simulink model "minseg_M2V3_2017a"  (R2017a)
settings: Solver=FixedStepDiscrete  StartTime=0.0  StopTime=inf  FixedStep=mdl_T_sample  RelTol=1e-3
undefined symbols (not defined in the file or in its folder): ctrl_lqr_K2, ctrl_motorDriver_v_ff_cmd_v_val, ctrl_motorDriver_v_ff_cmd_v_val_norm_dx_max, ctrl_motorDriver_v_ff_cmd_v_val_norm_dx_min, ctrl_motorDriver_v_output_max, ctrl_motorDriver_v_output_min, ctrl_motorDriver_v_pid_cmd_thetaDot_val, ctrl_motorDriver_v_pid_cmd_thetaDot_val_norm_dx_max, ctrl_motorDriver_v_pid_cmd_thetaDot_val_norm_dx_min, ctrl_motorDriver_v_pid_int_maxVal, ctrl_motorDriver_v_pid_int_minVal, ctrl_motorDriver_v_pid_k_d, ctrl_motorDriver_v_pid_k_i, ctrl_motorDriver_v_pid_k_p, ctrl_motorDriver_v_rts_ss_k_A, ctrl_motorDriver_v_rts_ss_k_B, ctrl_motorDriver_v_rts_ss_k_C, ctrl_motorDriver_v_rts_ss_k_D, ctrl_motorDriver_v_rts_ss_stateIC, ctrl_motorDriver_v_sfr_cmd_p_x_f, ctrl_motorDriver_v_sfr_cmd_p_x_mag, ctrl_motorDriver_v_sfr_cmd_p_y_f, ctrl_motorDriver_v_sfr_cmd_p_y_mag, ctrl_motorDriver_v_sfr_K, ctrl_motorDriver_v_sfr_K_plant, ctrl_motorDriver_v_sfr_K_rts, ctrl_motorDriver_v_T_cmd, ctrl_motorDriver_v_T_init, DiscIntNeverNeededParam, gyro_bias, io_srl_read_rateTransition_initialCondition, k_intmax_uint8, mdl_T_sample, mtr_encoder_filter_z_ss_A, mtr_encoder_filter_z_ss_B, mtr_encoder_filter_z_ss_C, mtr_encoder_filter_z_ss_D, plant, plant_accel_k_digital2analog, plant_body_l_c, plant_body_l_w, plant_gyro_encoder_filter_z_den, plant_gyro_encoder_filter_z_num, plant_gyro_filter_z_den, plant_gyro_filter_z_num, plant_gyro_k_digital2analog, plant_linear_ss_stateIC, plant_linear_ss_t_A, plant_linear_ss_t_B, plant_linear_ss_t_C, plant_linear_ss_t_D, plant_mtr_encoder_count2wheelRad, plant_mtr_encoder_filter_z_den, plant_mtr_encoder_filter_z_num, plant_pSupply_v, plant_supply_v, plant_T_init, plant_wheel_r
undefined symbols (not defined in the file): ctrl_lqr_addlDyn_A_discrete, ctrl_lqr_addlDyn_B_discrete, ctrl_lqr_addlDyn_C_discrete, ctrl_lqr_addlDyn_D_discrete, ctrl_lqr_addlDyn_k_antiWindup, ctrl_lqr_addlDyn_stateIC, plant_gyro_bias_movingAverage_n_pts, plant_linear_A_continuous, plant_linear_B_continuous, plant_linear_C_continuous, plant_linear_D_continuous, plant_linear_stateIC
libraries: svdutilitieslib x135, simulink x57, arduinolib x15, MinSegLibrary_M2V3 x3, dspindex x3, RASPlib x2
(part 4 of 6)

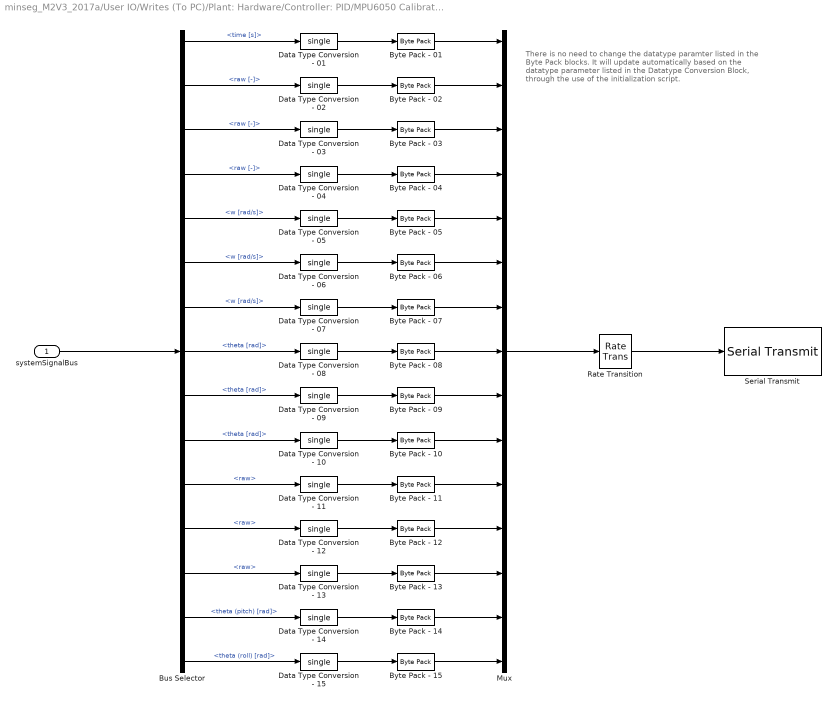
== system minseg_M2V3_2017a/User IO/Writes (To PC)/Plant: Hardware/Controller: PID/MPU6050 Calibration ==
  note: There is no need to change the datatype paramter
      | listed in the Byte Pack blocks.
      |
      | It will update automatically based on the datatype parameter
      | listed in the Datatype Conversion Block,
      | through the use of the initialization script.
  systemSignalBus : Inport
  Bus Selector : BusSelector  OutputSignals=plant.clock.time [s],plant.gyroscope.x.raw [-],plant.gyroscope.y.raw [-],plant.gyroscope.z.raw [-],plant.gyroscope.x.w [rad/s],plant.gyroscope.y.w [rad/s],plant.gyroscope.z.w [rad/s],plant.gyroscope.x.theta [rad],plant.gyroscope.y.theta [rad],plant.gyroscope.z.theta [rad],plant.accelerometer.x.raw,plant.accelerometer.y.raw,plant.accelerometer.z.raw,plant.accelerometer.x.theta (pitch) [rad],plant.accelerometer.z.theta (roll) [rad]
  Byte Pack - 01 : svdutilitieslib/Byte Pack  datatypes={'single'}  byteAlign=1  blockPlatform=arduinoert
      settings: AttributesFormatString=%<datatypes>  SourceProductName=Simulink Support Package for Arduino Hardware
  Byte Pack - 02 : svdutilitieslib/Byte Pack  datatypes={'single'}  byteAlign=1  blockPlatform=arduinoert
      settings: AttributesFormatString=%<datatypes>  SourceProductName=Simulink Support Package for Arduino Hardware
  Byte Pack - 03 : svdutilitieslib/Byte Pack  datatypes={'single'}  byteAlign=1  blockPlatform=arduinoert
      settings: AttributesFormatString=%<datatypes>  SourceProductName=Simulink Support Package for Arduino Hardware
  Byte Pack - 04 : svdutilitieslib/Byte Pack  datatypes={'single'}  byteAlign=1  blockPlatform=arduinoert
      settings: AttributesFormatString=%<datatypes>  SourceProductName=Simulink Support Package for Arduino Hardware
  Byte Pack - 05 : svdutilitieslib/Byte Pack  datatypes={'single'}  byteAlign=1  blockPlatform=arduinoert
      settings: AttributesFormatString=%<datatypes>  SourceProductName=Simulink Support Package for Arduino Hardware
  Byte Pack - 06 : svdutilitieslib/Byte Pack  datatypes={'single'}  byteAlign=1  blockPlatform=arduinoert
      settings: AttributesFormatString=%<datatypes>  SourceProductName=Simulink Support Package for Arduino Hardware
  Byte Pack - 07 : svdutilitieslib/Byte Pack  datatypes={'single'}  byteAlign=1  blockPlatform=arduinoert
      settings: AttributesFormatString=%<datatypes>  SourceProductName=Simulink Support Package for Arduino Hardware
  Byte Pack - 08 : svdutilitieslib/Byte Pack  datatypes={'single'}  byteAlign=1  blockPlatform=arduinoert
      settings: AttributesFormatString=%<datatypes>  SourceProductName=Simulink Support Package for Arduino Hardware
  Byte Pack - 09 : svdutilitieslib/Byte Pack  datatypes={'single'}  byteAlign=1  blockPlatform=arduinoert
      settings: AttributesFormatString=%<datatypes>  SourceProductName=Simulink Support Package for Arduino Hardware
  Byte Pack - {10..15} (6 alike) : svdutilitieslib/Byte Pack  datatypes={'single'}  byteAlign=1  blockPlatform=arduinoert
      settings: AttributesFormatString=%<datatypes>  SourceProductName=Simulink Support Package for Arduino Hardware
  Data Type Conversion - 01 : DataTypeConversion  OutDataTypeStr=single
  Data Type Conversion - 02 : DataTypeConversion  OutDataTypeStr=single
  Data Type Conversion - 03 : DataTypeConversion  OutDataTypeStr=single
  Data Type Conversion - 04 : DataTypeConversion  OutDataTypeStr=single
  Data Type Conversion - 05 : DataTypeConversion  OutDataTypeStr=single
  Data Type Conversion - 06 : DataTypeConversion  OutDataTypeStr=single
  Data Type Conversion - 07 : DataTypeConversion  OutDataTypeStr=single
  Data Type Conversion - 08 : DataTypeConversion  OutDataTypeStr=single
  Data Type Conversion - 09 : DataTypeConversion  OutDataTypeStr=single
  Data Type Conversion - {10..15} (6 alike) : DataTypeConversion  OutDataTypeStr=single
  Mux : Mux  Inputs=15
  Rate Transition : RateTransition  X0=io_srl_read_rateTransition_initialCondition  OutPortSampleTimeMultiple=io_read_rateTransition_decimation  OutPortSampleTime=io_srl_read_rateTransition_T_sample
      settings: AttributesFormatString=|
      | Output sample time: %<OutPortSampleTime>
      | Initial condition: %<X0>
  Serial Transmit : arduinolib/Serial Transmit  portNumber=0  sendmode=write  sendformat=Decimal  floatprecision=2  blockPlatform=arduino
      settings: SourceProductName=Simulink Support Package for Arduino Hardware
  wires:
  Byte Pack - 04/1 -> Mux/4
  Byte Pack - 03/1 -> Mux/3
  Byte Pack - 07/1 -> Mux/7
  Mux/1 -> Rate Transition/1
  Byte Pack - 01/1 -> Mux/1
  Byte Pack - 06/1 -> Mux/6
  Byte Pack - 05/1 -> Mux/5
  Byte Pack - 08/1 -> Mux/8
  Byte Pack - 02/1 -> Mux/2
  systemSignalBus/1 -> Bus Selector/1
  Byte Pack - 09/1 -> Mux/9
  Byte Pack - 10/1 -> Mux/10
  Data Type Conversion - 01/1 -> Byte Pack - 01/1
  Data Type Conversion - 02/1 -> Byte Pack - 02/1
  Data Type Conversion - 03/1 -> Byte Pack - 03/1
  Data Type Conversion - 04/1 -> Byte Pack - 04/1
  Data Type Conversion - 05/1 -> Byte Pack - 05/1
  Data Type Conversion - 06/1 -> Byte Pack - 06/1
  Data Type Conversion - 07/1 -> Byte Pack - 07/1
  Data Type Conversion - 08/1 -> Byte Pack - 08/1
  Data Type Conversion - 09/1 -> Byte Pack - 09/1
  Data Type Conversion - 10/1 -> Byte Pack - 10/1
  Rate Transition/1 -> Serial Transmit/1
  Bus Selector/1 -> Data Type Conversion - 01/1  "<time [s]>"
  Data Type Conversion - 11/1 -> Byte Pack - 11/1
  Data Type Conversion - 12/1 -> Byte Pack - 12/1
  Data Type Conversion - 13/1 -> Byte Pack - 13/1
  Data Type Conversion - 14/1 -> Byte Pack - 14/1
  Data Type Conversion - 15/1 -> Byte Pack - 15/1
  Byte Pack - 11/1 -> Mux/11
  Byte Pack - 12/1 -> Mux/12
  Byte Pack - 13/1 -> Mux/13
  Byte Pack - 14/1 -> Mux/14
  Byte Pack - 15/1 -> Mux/15
  Bus Selector/2 -> Data Type Conversion - 02/1  "<raw [-]>"
  Bus Selector/3 -> Data Type Conversion - 03/1  "<raw [-]>"
  Bus Selector/4 -> Data Type Conversion - 04/1  "<raw [-]>"
  Bus Selector/5 -> Data Type Conversion - 05/1  "<w [rad/s]>"
  Bus Selector/6 -> Data Type Conversion - 06/1  "<w [rad/s]>"
  Bus Selector/7 -> Data Type Conversion - 07/1  "<w [rad/s]>"
  Bus Selector/8 -> Data Type Conversion - 08/1  "<theta [rad]>"
  Bus Selector/11 -> Data Type Conversion - 11/1  "<raw>"
  Bus Selector/12 -> Data Type Conversion - 12/1  "<raw>"
  Bus Selector/9 -> Data Type Conversion - 09/1  "<theta [rad]>"
  Bus Selector/10 -> Data Type Conversion - 10/1  "<theta [rad]>"
  Bus Selector/13 -> Data Type Conversion - 13/1  "<raw>"
  Bus Selector/14 -> Data Type Conversion - 14/1  "<theta (pitch) [rad]>"
  Bus Selector/15 -> Data Type Conversion - 15/1  "<theta (roll) [rad]>"

== system minseg_M2V3_2017a/User IO/Writes (To PC)/Plant: Hardware/Controller: PID/Standard ==
  note: There is no need to change the datatype parameter
      | listed in the Byte Pack blocks.
      |
      | It will update automatically based on the datatype parameter
      | listed in the Datatype Conversion Block,
      | through the use of the initialization script.
  systemSignalBus : Inport
  Bus Selector : BusSelector  OutputSignals=clock.time [s],userIO.read.controller.command.left.theta_global_average_dot [rad/s],controller.v_motorDriver.output.left.command [V].saturated,controller.v_motorDriver.output.middle.command [V].saturated,plant.state.wheel_angularPosition_theta_global_average [rad],plant.state.body_angularPosition_phi_x [rad],plant.state.wheel_angularVelocity_thetaDot_global_average [rad/s],plant.state.body_angularVelocity_phiDot_x [rad/s],plant.state.body_angularPosition_phi_y [rad],plant.state.body_angularVelocity_phiDot_y [rad/s]
  Byte Pack - 01 : svdutilitieslib/Byte Pack  datatypes={'single'}  byteAlign=1  blockPlatform=arduinoert
      settings: AttributesFormatString=%<datatypes>  SourceProductName=Simulink Support Package for Arduino Hardware
  Byte Pack - 02 : svdutilitieslib/Byte Pack  datatypes={'single'}  byteAlign=1  blockPlatform=arduinoert
      settings: AttributesFormatString=%<datatypes>  SourceProductName=Simulink Support Package for Arduino Hardware
  Byte Pack - 03 : svdutilitieslib/Byte Pack  datatypes={'single'}  byteAlign=1  blockPlatform=arduinoert
      settings: AttributesFormatString=%<datatypes>  SourceProductName=Simulink Support Package for Arduino Hardware
  Byte Pack - 04 : svdutilitieslib/Byte Pack  datatypes={'single'}  byteAlign=1  blockPlatform=arduinoert
      settings: AttributesFormatString=%<datatypes>  SourceProductName=Simulink Support Package for Arduino Hardware
  Byte Pack - 05 : svdutilitieslib/Byte Pack  datatypes={'single'}  byteAlign=1  blockPlatform=arduinoert
      settings: AttributesFormatString=%<datatypes>  SourceProductName=Simulink Support Package for Arduino Hardware
  Byte Pack - 06 : svdutilitieslib/Byte Pack  datatypes={'single'}  byteAlign=1  blockPlatform=arduinoert
      settings: AttributesFormatString=%<datatypes>  SourceProductName=Simulink Support Package for Arduino Hardware
  Byte Pack - 07 : svdutilitieslib/Byte Pack  datatypes={'single'}  byteAlign=1  blockPlatform=arduinoert
      settings: AttributesFormatString=%<datatypes>  SourceProductName=Simulink Support Package for Arduino Hardware
  Byte Pack - 08 : svdutilitieslib/Byte Pack  datatypes={'single'}  byteAlign=1  blockPlatform=arduinoert
      settings: AttributesFormatString=%<datatypes>  SourceProductName=Simulink Support Package for Arduino Hardware
  Byte Pack - 09 : svdutilitieslib/Byte Pack  datatypes={'single'}  byteAlign=1  blockPlatform=arduinoert
      settings: AttributesFormatString=%<datatypes>  SourceProductName=Simulink Support Package for Arduino Hardware
  Byte Pack - 10 : svdutilitieslib/Byte Pack  datatypes={'single'}  byteAlign=1  blockPlatform=arduinoert
      settings: AttributesFormatString=%<datatypes>  SourceProductName=Simulink Support Package for Arduino Hardware
  Data Type Conversion - 01 : DataTypeConversion  OutDataTypeStr=single
  Data Type Conversion - 02 : DataTypeConversion  OutDataTypeStr=single
  Data Type Conversion - 03 : DataTypeConversion  OutDataTypeStr=single
  Data Type Conversion - 04 : DataTypeConversion  OutDataTypeStr=single
  Data Type Conversion - 05 : DataTypeConversion  OutDataTypeStr=single
  Data Type Conversion - 06 : DataTypeConversion  OutDataTypeStr=single
  Data Type Conversion - 07 : DataTypeConversion  OutDataTypeStr=single
  Data Type Conversion - 08 : DataTypeConversion  OutDataTypeStr=single
  Data Type Conversion - 09 : DataTypeConversion  OutDataTypeStr=single
  Data Type Conversion - 10 : DataTypeConversion  OutDataTypeStr=single
  Mux : Mux  Inputs=10
  Rate Transition : RateTransition  X0=0 %io_srl_read_rateTransition_initialCondition  OutPortSampleTimeMultiple=io_read_rateTransition_decimation  OutPortSampleTime=io_srl_read_rateTransition_T_sample
      settings: AttributesFormatString=|
      | Output sample time: %<OutPortSampleTime>
      | Initial condition: %<X0>
  Serial Transmit : arduinolib/Serial Transmit  portNumber=srl_port  sendmode=write  sendformat=Decimal  floatprecision=2  blockPlatform=arduino
      settings: SourceProductName=Simulink Support Package for Arduino Hardware
  wires:
  Mux/1 -> Serial Transmit/1
  Data Type Conversion - 10/1 -> Byte Pack - 10/1
  Data Type Conversion - 09/1 -> Byte Pack - 09/1
  Data Type Conversion - 08/1 -> Byte Pack - 08/1
  Data Type Conversion - 07/1 -> Byte Pack - 07/1
  Data Type Conversion - 06/1 -> Byte Pack - 06/1
  Data Type Conversion - 05/1 -> Byte Pack - 05/1
  Data Type Conversion - 04/1 -> Byte Pack - 04/1
  Data Type Conversion - 03/1 -> Byte Pack - 03/1
  Data Type Conversion - 02/1 -> Byte Pack - 02/1
  Data Type Conversion - 01/1 -> Byte Pack - 01/1
  Byte Pack - 10/1 -> Mux/10
  Byte Pack - 09/1 -> Mux/9
  systemSignalBus/1 -> Rate Transition/1
  Byte Pack - 02/1 -> Mux/2
  Byte Pack - 08/1 -> Mux/8
  Byte Pack - 05/1 -> Mux/5
  Byte Pack - 06/1 -> Mux/6
  Byte Pack - 01/1 -> Mux/1
  Byte Pack - 07/1 -> Mux/7
  Byte Pack - 03/1 -> Mux/3
  Byte Pack - 04/1 -> Mux/4
  Bus Selector/1 -> Data Type Conversion - 01/1  "<time [s]>"
  Bus Selector/2 -> Data Type Conversion - 02/1  "<theta_global_average_dot [rad/s]>"
  Bus Selector/3 -> Data Type Conversion - 03/1  "<saturated>"
  Bus Selector/4 -> Data Type Conversion - 04/1  "<saturated>"
  Bus Selector/5 -> Data Type Conversion - 05/1  "<wheel_angularPosition_theta_global_average [rad]>"
  Bus Selector/6 -> Data Type Conversion - 06/1  "<body_angularPosition_phi_x [rad]>"
  Bus Selector/7 -> Data Type Conversion - 07/1  "<wheel_angularVelocity_thetaDot_global_average [rad/s]>"
  Bus Selector/8 -> Data Type Conversion - 08/1  "<body_angularVelocity_phiDot_x [rad/s]>"
  Bus Selector/9 -> Data Type Conversion - 09/1  "<body_angularPosition_phi_y [rad]>"
  Bus Selector/10 -> Data Type Conversion - 10/1  "<body_angularVelocity_phiDot_y [rad/s]>"
  Rate Transition/1 -> Bus Selector/1

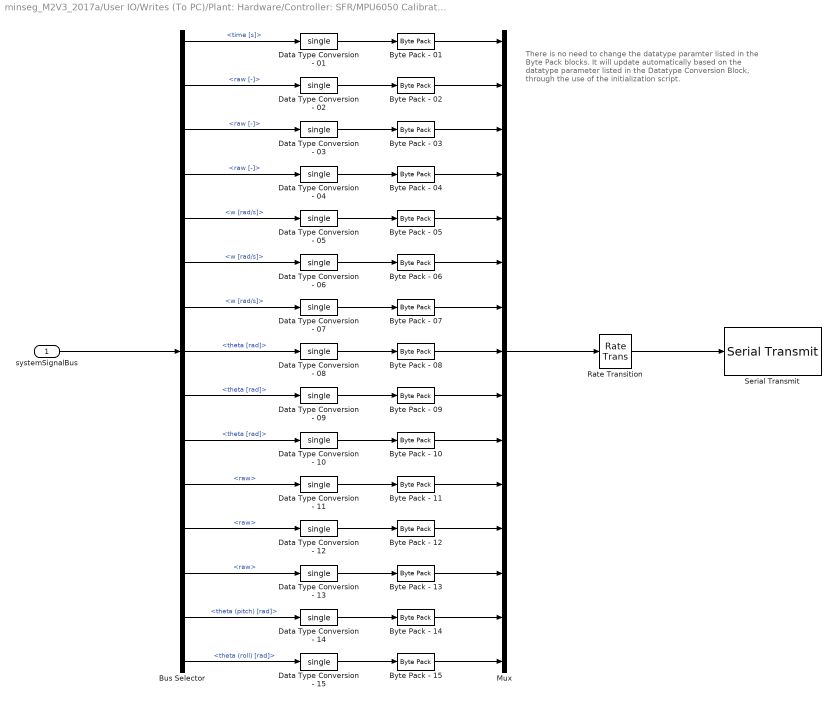
== system minseg_M2V3_2017a/User IO/Writes (To PC)/Plant: Hardware/Controller: SFR/MPU6050 Calibration ==
  note: There is no need to change the datatype paramter
      | listed in the Byte Pack blocks.
      |
      | It will update automatically based on the datatype parameter
      | listed in the Datatype Conversion Block,
      | through the use of the initialization script.
  systemSignalBus : Inport
  Bus Selector : BusSelector  OutputSignals=plant.clock.time [s],plant.gyroscope.x.raw [-],plant.gyroscope.y.raw [-],plant.gyroscope.z.raw [-],plant.gyroscope.x.w [rad/s],plant.gyroscope.y.w [rad/s],plant.gyroscope.z.w [rad/s],plant.gyroscope.x.theta [rad],plant.gyroscope.y.theta [rad],plant.gyroscope.z.theta [rad],plant.accelerometer.x.raw,plant.accelerometer.y.raw,plant.accelerometer.z.raw,plant.accelerometer.x.theta (pitch) [rad],plant.accelerometer.z.theta (roll) [rad]
  Byte Pack - 01 : svdutilitieslib/Byte Pack  datatypes={'single'}  byteAlign=1  blockPlatform=arduinoert
      settings: AttributesFormatString=%<datatypes>  SourceProductName=Simulink Support Package for Arduino Hardware
  Byte Pack - 02 : svdutilitieslib/Byte Pack  datatypes={'single'}  byteAlign=1  blockPlatform=arduinoert
      settings: AttributesFormatString=%<datatypes>  SourceProductName=Simulink Support Package for Arduino Hardware
  Byte Pack - 03 : svdutilitieslib/Byte Pack  datatypes={'single'}  byteAlign=1  blockPlatform=arduinoert
      settings: AttributesFormatString=%<datatypes>  SourceProductName=Simulink Support Package for Arduino Hardware
  Byte Pack - 04 : svdutilitieslib/Byte Pack  datatypes={'single'}  byteAlign=1  blockPlatform=arduinoert
      settings: AttributesFormatString=%<datatypes>  SourceProductName=Simulink Support Package for Arduino Hardware
  Byte Pack - 05 : svdutilitieslib/Byte Pack  datatypes={'single'}  byteAlign=1  blockPlatform=arduinoert
      settings: AttributesFormatString=%<datatypes>  SourceProductName=Simulink Support Package for Arduino Hardware
  Byte Pack - 06 : svdutilitieslib/Byte Pack  datatypes={'single'}  byteAlign=1  blockPlatform=arduinoert
      settings: AttributesFormatString=%<datatypes>  SourceProductName=Simulink Support Package for Arduino Hardware
  Byte Pack - 07 : svdutilitieslib/Byte Pack  datatypes={'single'}  byteAlign=1  blockPlatform=arduinoert
      settings: AttributesFormatString=%<datatypes>  SourceProductName=Simulink Support Package for Arduino Hardware
  Byte Pack - 08 : svdutilitieslib/Byte Pack  datatypes={'single'}  byteAlign=1  blockPlatform=arduinoert
      settings: AttributesFormatString=%<datatypes>  SourceProductName=Simulink Support Package for Arduino Hardware
  Byte Pack - 09 : svdutilitieslib/Byte Pack  datatypes={'single'}  byteAlign=1  blockPlatform=arduinoert
      settings: AttributesFormatString=%<datatypes>  SourceProductName=Simulink Support Package for Arduino Hardware
  Byte Pack - {10..15} (6 alike) : svdutilitieslib/Byte Pack  datatypes={'single'}  byteAlign=1  blockPlatform=arduinoert
      settings: AttributesFormatString=%<datatypes>  SourceProductName=Simulink Support Package for Arduino Hardware
  Data Type Conversion - 01 : DataTypeConversion  OutDataTypeStr=single
  Data Type Conversion - 02 : DataTypeConversion  OutDataTypeStr=single
  Data Type Conversion - 03 : DataTypeConversion  OutDataTypeStr=single
  Data Type Conversion - 04 : DataTypeConversion  OutDataTypeStr=single
  Data Type Conversion - 05 : DataTypeConversion  OutDataTypeStr=single
  Data Type Conversion - 06 : DataTypeConversion  OutDataTypeStr=single
  Data Type Conversion - 07 : DataTypeConversion  OutDataTypeStr=single
  Data Type Conversion - 08 : DataTypeConversion  OutDataTypeStr=single
  Data Type Conversion - 09 : DataTypeConversion  OutDataTypeStr=single
  Data Type Conversion - {10..15} (6 alike) : DataTypeConversion  OutDataTypeStr=single
  Mux : Mux  Inputs=15
  Rate Transition : RateTransition  X0=io_srl_read_rateTransition_initialCondition  OutPortSampleTimeMultiple=io_read_rateTransition_decimation  OutPortSampleTime=io_srl_read_rateTransition_T_sample
      settings: AttributesFormatString=|
      | Output sample time: %<OutPortSampleTime>
      | Initial condition: %<X0>
  Serial Transmit : arduinolib/Serial Transmit  portNumber=0  sendmode=write  sendformat=Decimal  floatprecision=2  blockPlatform=arduino
      settings: SourceProductName=Simulink Support Package for Arduino Hardware
  wires:
  Bus Selector/15 -> Data Type Conversion - 15/1  "<theta (roll) [rad]>"
  Bus Selector/14 -> Data Type Conversion - 14/1  "<theta (pitch) [rad]>"
  Bus Selector/13 -> Data Type Conversion - 13/1  "<raw>"
  Bus Selector/10 -> Data Type Conversion - 10/1  "<theta [rad]>"
  Bus Selector/9 -> Data Type Conversion - 09/1  "<theta [rad]>"
  Bus Selector/12 -> Data Type Conversion - 12/1  "<raw>"
  Bus Selector/11 -> Data Type Conversion - 11/1  "<raw>"
  Bus Selector/8 -> Data Type Conversion - 08/1  "<theta [rad]>"
  Bus Selector/7 -> Data Type Conversion - 07/1  "<w [rad/s]>"
  Bus Selector/6 -> Data Type Conversion - 06/1  "<w [rad/s]>"
  Bus Selector/5 -> Data Type Conversion - 05/1  "<w [rad/s]>"
  Bus Selector/4 -> Data Type Conversion - 04/1  "<raw [-]>"
  Bus Selector/3 -> Data Type Conversion - 03/1  "<raw [-]>"
  Bus Selector/2 -> Data Type Conversion - 02/1  "<raw [-]>"
  Byte Pack - 15/1 -> Mux/15
  Byte Pack - 14/1 -> Mux/14
  Byte Pack - 13/1 -> Mux/13
  Byte Pack - 12/1 -> Mux/12
  Byte Pack - 11/1 -> Mux/11
  Data Type Conversion - 15/1 -> Byte Pack - 15/1
  Data Type Conversion - 14/1 -> Byte Pack - 14/1
  Data Type Conversion - 13/1 -> Byte Pack - 13/1
  Data Type Conversion - 12/1 -> Byte Pack - 12/1
  Data Type Conversion - 11/1 -> Byte Pack - 11/1
  Bus Selector/1 -> Data Type Conversion - 01/1  "<time [s]>"
  Rate Transition/1 -> Serial Transmit/1
  Data Type Conversion - 10/1 -> Byte Pack - 10/1
  Data Type Conversion - 09/1 -> Byte Pack - 09/1
  Data Type Conversion - 08/1 -> Byte Pack - 08/1
  Data Type Conversion - 07/1 -> Byte Pack - 07/1
  Data Type Conversion - 06/1 -> Byte Pack - 06/1
  Data Type Conversion - 05/1 -> Byte Pack - 05/1
  Data Type Conversion - 04/1 -> Byte Pack - 04/1
  Data Type Conversion - 03/1 -> Byte Pack - 03/1
  Data Type Conversion - 02/1 -> Byte Pack - 02/1
  Data Type Conversion - 01/1 -> Byte Pack - 01/1
  Byte Pack - 10/1 -> Mux/10
  Byte Pack - 09/1 -> Mux/9
  systemSignalBus/1 -> Bus Selector/1
  Byte Pack - 02/1 -> Mux/2
  Byte Pack - 08/1 -> Mux/8
  Byte Pack - 05/1 -> Mux/5
  Byte Pack - 06/1 -> Mux/6
  Byte Pack - 01/1 -> Mux/1
  Mux/1 -> Rate Transition/1
  Byte Pack - 07/1 -> Mux/7
  Byte Pack - 03/1 -> Mux/3
  Byte Pack - 04/1 -> Mux/4

== system minseg_M2V3_2017a/User IO/Writes (To PC)/Plant: Hardware/Controller: SFR/Motor Characterization ==
  note: There is no need to change the datatype paramter
      | listed in the Byte Pack blocks.
      |
      | It will update automatically based on the datatype parameter
      | listed in the Datatype Conversion Block,
      | through the use of the initialization script.
  systemSignalBus : Inport
  Bus Selector : BusSelector  OutputSignals="plant.clock.time [s],io.reads.userInput.controller.output_vMotor.command,plant.encoders.left.angularVelocity  [rad/s],plant.encoders.middle.angularVelocity  [rad/s],controller.motorAngularVelocity.left.voltage.command [V],controller.motorAngularVelocity.middle.voltage.command [V],plant.drivers.left.voltage.command.digital.positive [V],plant.drivers.left.voltage.command.digital.negative [V],plant.drivers.middle.voltage.command.digital.positive [V],plant.drivers.middle.voltage.command.digital.negative [V]"
  Byte Pack - 01 : svdutilitieslib/Byte Pack  datatypes={'single'}  byteAlign=1  blockPlatform=arduinoert
      settings: AttributesFormatString=%<datatypes>  SourceProductName=Simulink Support Package for Arduino Hardware
  Byte Pack - 02 : svdutilitieslib/Byte Pack  datatypes={'single'}  byteAlign=1  blockPlatform=arduinoert
      settings: AttributesFormatString=%<datatypes>  SourceProductName=Simulink Support Package for Arduino Hardware
  Byte Pack - 03 : svdutilitieslib/Byte Pack  datatypes={'single'}  byteAlign=1  blockPlatform=arduinoert
      settings: AttributesFormatString=%<datatypes>  SourceProductName=Simulink Support Package for Arduino Hardware
  Byte Pack - 04 : svdutilitieslib/Byte Pack  datatypes={'single'}  byteAlign=1  blockPlatform=arduinoert
      settings: AttributesFormatString=%<datatypes>  SourceProductName=Simulink Support Package for Arduino Hardware
  Byte Pack - 05 : svdutilitieslib/Byte Pack  datatypes={'single'}  byteAlign=1  blockPlatform=arduinoert
      settings: AttributesFormatString=%<datatypes>  SourceProductName=Simulink Support Package for Arduino Hardware
  Byte Pack - 06 : svdutilitieslib/Byte Pack  datatypes={'single'}  byteAlign=1  blockPlatform=arduinoert
      settings: AttributesFormatString=%<datatypes>  SourceProductName=Simulink Support Package for Arduino Hardware
  Byte Pack - 07 : svdutilitieslib/Byte Pack  datatypes={'single'}  byteAlign=1  blockPlatform=arduinoert
      settings: AttributesFormatString=%<datatypes>  SourceProductName=Simulink Support Package for Arduino Hardware
  Byte Pack - 08 : svdutilitieslib/Byte Pack  datatypes={'single'}  byteAlign=1  blockPlatform=arduinoert
      settings: AttributesFormatString=%<datatypes>  SourceProductName=Simulink Support Package for Arduino Hardware
  Byte Pack - 09 : svdutilitieslib/Byte Pack  datatypes={'uint8'}  byteAlign=1  blockPlatform=arduinoert
      settings: AttributesFormatString=%<datatypes>  SourceProductName=Simulink Support Package for Arduino Hardware
  Byte Pack - 10 : svdutilitieslib/Byte Pack  datatypes={'uint8'}  byteAlign=1  blockPlatform=arduinoert
      settings: AttributesFormatString=%<datatypes>  SourceProductName=Simulink Support Package for Arduino Hardware
  Data Type Conversion - 01 : DataTypeConversion  OutDataTypeStr=single
  Data Type Conversion - 02 : DataTypeConversion  OutDataTypeStr=single
  Data Type Conversion - 03 : DataTypeConversion  OutDataTypeStr=single
  Data Type Conversion - 04 : DataTypeConversion  OutDataTypeStr=single
  Data Type Conversion - 05 : DataTypeConversion  OutDataTypeStr=single
  Data Type Conversion - 06 : DataTypeConversion  OutDataTypeStr=single
  Data Type Conversion - 07 : DataTypeConversion  OutDataTypeStr=uint8
  Data Type Conversion - 08 : DataTypeConversion  OutDataTypeStr=uint8
  Data Type Conversion - 09 : DataTypeConversion  OutDataTypeStr=uint8
  Data Type Conversion - 10 : DataTypeConversion  OutDataTypeStr=uint8
  Mux : Mux  Inputs=10
  Rate Transition : RateTransition  X0=io_srl_read_rateTransition_initialCondition  OutPortSampleTimeMultiple=io_read_rateTransition_decimation  OutPortSampleTime=io_srl_read_rateTransition_T_sample
      settings: AttributesFormatString=|
      | Output sample time: %<OutPortSampleTime>
      | Initial condition: %<X0>
  Serial Transmit : arduinolib/Serial Transmit  portNumber=0  sendmode=write  sendformat=Decimal  floatprecision=2  blockPlatform=arduino
      settings: SourceProductName=Simulink Support Package for Arduino Hardware
  wires:
  Bus Selector/10 -> Data Type Conversion - 10/1  "<negative [V]>"
  Bus Selector/9 -> Data Type Conversion - 09/1  "<positive [V]>"
  Bus Selector/8 -> Data Type Conversion - 08/1  "<negative [V]>"
  Bus Selector/7 -> Data Type Conversion - 07/1  "<positive [V]>"
  Bus Selector/6 -> Data Type Conversion - 06/1  "<command [V]>"
  Bus Selector/5 -> Data Type Conversion - 05/1  "<command [V]>"
  Byte Pack - 04/1 -> Mux/4
  Byte Pack - 03/1 -> Mux/3
  Byte Pack - 07/1 -> Mux/7
  Mux/1 -> Rate Transition/1
  Byte Pack - 01/1 -> Mux/1
  Byte Pack - 06/1 -> Mux/6
  Byte Pack - 05/1 -> Mux/5
  Byte Pack - 08/1 -> Mux/8
  Byte Pack - 02/1 -> Mux/2
  systemSignalBus/1 -> Bus Selector/1
  Bus Selector/2 -> Data Type Conversion - 02/1  "<command>"
  Byte Pack - 09/1 -> Mux/9
  Byte Pack - 10/1 -> Mux/10
  Data Type Conversion - 01/1 -> Byte Pack - 01/1
  Data Type Conversion - 02/1 -> Byte Pack - 02/1
  Data Type Conversion - 03/1 -> Byte Pack - 03/1
  Data Type Conversion - 04/1 -> Byte Pack - 04/1
  Data Type Conversion - 05/1 -> Byte Pack - 05/1
  Data Type Conversion - 06/1 -> Byte Pack - 06/1
  Data Type Conversion - 07/1 -> Byte Pack - 07/1
  Data Type Conversion - 08/1 -> Byte Pack - 08/1
  Data Type Conversion - 09/1 -> Byte Pack - 09/1
  Data Type Conversion - 10/1 -> Byte Pack - 10/1
  Bus Selector/3 -> Data Type Conversion - 03/1  "<angularVelocity  [rad/s]>"
  Bus Selector/4 -> Data Type Conversion - 04/1  "<angularVelocity  [rad/s]>"
  Rate Transition/1 -> Serial Transmit/1
  Bus Selector/1 -> Data Type Conversion - 01/1  "<time [s]>"

== system minseg_M2V3_2017a/User IO/Writes (To PC)/Plant: Hardware/Controller: SFR/Standard ==
  note: There is no need to change the datatype parameter
      | listed in the Byte Pack blocks.
      |
      | It will update automatically based on the datatype parameter
      | listed in the Datatype Conversion Block,
      | through the use of the initialization script.
  systemSignalBus : Inport
  Bus Selector : BusSelector  OutputSignals=clock.time [s],controller.v_motorDriver.output.left.command [V].saturated,controller.v_motorDriver.output.middle.command [V].saturated,plant.position.phi.x (pitch).position [rad],userIO.read.controller.command.theta_global_average [rad],plant.position.theta.global.average.position [rad],userIO.read.controller.command.phi_y [rad],plant.position.phi.y (yaw).position [rad],plant.position.theta.global.average.velocity [rad/s],plant.position.phi.x (pitch).velocity [rad/s]
  Byte Pack - 01 : svdutilitieslib/Byte Pack  datatypes={'single'}  byteAlign=1  blockPlatform=arduinoert
      settings: AttributesFormatString=%<datatypes>  SourceProductName=Simulink Support Package for Arduino Hardware
  Byte Pack - 02 : svdutilitieslib/Byte Pack  datatypes={'single'}  byteAlign=1  blockPlatform=arduinoert
      settings: AttributesFormatString=%<datatypes>  SourceProductName=Simulink Support Package for Arduino Hardware
  Byte Pack - 03 : svdutilitieslib/Byte Pack  datatypes={'single'}  byteAlign=1  blockPlatform=arduinoert
      settings: AttributesFormatString=%<datatypes>  SourceProductName=Simulink Support Package for Arduino Hardware
  Byte Pack - 04 : svdutilitieslib/Byte Pack  datatypes={'single'}  byteAlign=1  blockPlatform=arduinoert
      settings: AttributesFormatString=%<datatypes>  SourceProductName=Simulink Support Package for Arduino Hardware
  Byte Pack - 05 : svdutilitieslib/Byte Pack  datatypes={'single'}  byteAlign=1  blockPlatform=arduinoert
      settings: AttributesFormatString=%<datatypes>  SourceProductName=Simulink Support Package for Arduino Hardware
  Byte Pack - 06 : svdutilitieslib/Byte Pack  datatypes={'single'}  byteAlign=1  blockPlatform=arduinoert
      settings: AttributesFormatString=%<datatypes>  SourceProductName=Simulink Support Package for Arduino Hardware
  Byte Pack - 07 : svdutilitieslib/Byte Pack  datatypes={'single'}  byteAlign=1  blockPlatform=arduinoert
      settings: AttributesFormatString=%<datatypes>  SourceProductName=Simulink Support Package for Arduino Hardware
  Byte Pack - 08 : svdutilitieslib/Byte Pack  datatypes={'single'}  byteAlign=1  blockPlatform=arduinoert
      settings: AttributesFormatString=%<datatypes>  SourceProductName=Simulink Support Package for Arduino Hardware
  Byte Pack - 09 : svdutilitieslib/Byte Pack  datatypes={'single'}  byteAlign=1  blockPlatform=arduinoert
      settings: AttributesFormatString=%<datatypes>  SourceProductName=Simulink Support Package for Arduino Hardware
  Byte Pack - 10 : svdutilitieslib/Byte Pack  datatypes={'single'}  byteAlign=1  blockPlatform=arduinoert
      settings: AttributesFormatString=%<datatypes>  SourceProductName=Simulink Support Package for Arduino Hardware
  Data Type Conversion - 01 : DataTypeConversion  OutDataTypeStr=single
  Data Type Conversion - 02 : DataTypeConversion  OutDataTypeStr=single
  Data Type Conversion - 03 : DataTypeConversion  OutDataTypeStr=single
  Data Type Conversion - 04 : DataTypeConversion  OutDataTypeStr=single
  Data Type Conversion - 05 : DataTypeConversion  OutDataTypeStr=single
  Data Type Conversion - 06 : DataTypeConversion  OutDataTypeStr=single
  Data Type Conversion - 07 : DataTypeConversion  OutDataTypeStr=single
  Data Type Conversion - 08 : DataTypeConversion  OutDataTypeStr=single
  Data Type Conversion - 09 : DataTypeConversion  OutDataTypeStr=single
  Data Type Conversion - 10 : DataTypeConversion  OutDataTypeStr=single
  Mux : Mux  Inputs=10
  Rate Transition : RateTransition  X0=0 %io_srl_read_rateTransition_initialCondition  OutPortSampleTimeMultiple=io_read_rateTransition_decimation  OutPortSampleTime=io_srl_read_rateTransition_T_sample
      settings: AttributesFormatString=|
      | Output sample time: %<OutPortSampleTime>
      | Initial condition: %<X0>
  Serial Transmit : arduinolib/Serial Transmit  portNumber=srl_port  sendmode=write  sendformat=Decimal  floatprecision=2  blockPlatform=arduino
      settings: SourceProductName=Simulink Support Package for Arduino Hardware
  wires:
  Byte Pack - 04/1 -> Mux/4
  Byte Pack - 03/1 -> Mux/3
  Byte Pack - 07/1 -> Mux/7
  Byte Pack - 01/1 -> Mux/1
  Byte Pack - 06/1 -> Mux/6
  Byte Pack - 05/1 -> Mux/5
  Byte Pack - 08/1 -> Mux/8
  Byte Pack - 02/1 -> Mux/2
  systemSignalBus/1 -> Rate Transition/1
  Byte Pack - 09/1 -> Mux/9
  Byte Pack - 10/1 -> Mux/10
  Data Type Conversion - 01/1 -> Byte Pack - 01/1
  Data Type Conversion - 02/1 -> Byte Pack - 02/1
  Data Type Conversion - 03/1 -> Byte Pack - 03/1
  Data Type Conversion - 04/1 -> Byte Pack - 04/1
  Data Type Conversion - 05/1 -> Byte Pack - 05/1
  Data Type Conversion - 06/1 -> Byte Pack - 06/1
  Data Type Conversion - 07/1 -> Byte Pack - 07/1
  Data Type Conversion - 08/1 -> Byte Pack - 08/1
  Data Type Conversion - 09/1 -> Byte Pack - 09/1
  Data Type Conversion - 10/1 -> Byte Pack - 10/1
  Mux/1 -> Serial Transmit/1
  Bus Selector/1 -> Data Type Conversion - 01/1  "<time [s]>"
  Bus Selector/2 -> Data Type Conversion - 02/1  "<saturated>"
  Bus Selector/3 -> Data Type Conversion - 03/1  "<saturated>"
  Bus Selector/4 -> Data Type Conversion - 04/1  "<position [rad]>"
  Bus Selector/5 -> Data Type Conversion - 05/1  "<theta_global_average [rad]>"
  Bus Selector/6 -> Data Type Conversion - 06/1  "<position [rad]>"
  Bus Selector/7 -> Data Type Conversion - 07/1  "<phi_y [rad]>"
  Bus Selector/8 -> Data Type Conversion - 08/1  "<position [rad]>"
  Bus Selector/9 -> Data Type Conversion - 09/1  "<velocity [rad/s]>"
  Bus Selector/10 -> Data Type Conversion - 10/1  "<velocity [rad/s]>"
  Rate Transition/1 -> Bus Selector/1

== system minseg_M2V3_2017a/User IO/Writes (To PC)/Plant: Linear Dynamics/Controller: FF/Motor Characterization ==
  note: There is no need to change the datatype paramter
      | listed in the Byte Pack blocks.
      |
      | It will update automatically based on the datatype parameter
      | listed in the Datatype Conversion Block,
      | through the use of the initialization script.
  systemSignalBus : Inport
  Bus Selector : BusSelector  OutputSignals="plant.clock.time [s],io.reads.userInput.controller.output_vMotor.command,plant.encoders.left.angularVelocity  [rad/s],plant.encoders.middle.angularVelocity  [rad/s],controller.motorAngularVelocity.left.voltage.command [V],controller.motorAngularVelocity.middle.voltage.command [V],plant.drivers.left.voltage.command.digital.positive [V],plant.drivers.left.voltage.command.digital.negative [V],plant.drivers.middle.voltage.command.digital.positive [V],plant.drivers.middle.voltage.command.digital.negative [V]"
  Byte Pack - 01 : svdutilitieslib/Byte Pack  datatypes={'single'}  byteAlign=1  blockPlatform=arduinoert
      settings: AttributesFormatString=%<datatypes>  SourceProductName=Simulink Support Package for Arduino Hardware
  Byte Pack - 02 : svdutilitieslib/Byte Pack  datatypes={'single'}  byteAlign=1  blockPlatform=arduinoert
      settings: AttributesFormatString=%<datatypes>  SourceProductName=Simulink Support Package for Arduino Hardware
  Byte Pack - 03 : svdutilitieslib/Byte Pack  datatypes={'single'}  byteAlign=1  blockPlatform=arduinoert
      settings: AttributesFormatString=%<datatypes>  SourceProductName=Simulink Support Package for Arduino Hardware
  Byte Pack - 04 : svdutilitieslib/Byte Pack  datatypes={'single'}  byteAlign=1  blockPlatform=arduinoert
      settings: AttributesFormatString=%<datatypes>  SourceProductName=Simulink Support Package for Arduino Hardware
  Byte Pack - 05 : svdutilitieslib/Byte Pack  datatypes={'single'}  byteAlign=1  blockPlatform=arduinoert
      settings: AttributesFormatString=%<datatypes>  SourceProductName=Simulink Support Package for Arduino Hardware
  Byte Pack - 06 : svdutilitieslib/Byte Pack  datatypes={'single'}  byteAlign=1  blockPlatform=arduinoert
      settings: AttributesFormatString=%<datatypes>  SourceProductName=Simulink Support Package for Arduino Hardware
  Byte Pack - 07 : svdutilitieslib/Byte Pack  datatypes={'single'}  byteAlign=1  blockPlatform=arduinoert
      settings: AttributesFormatString=%<datatypes>  SourceProductName=Simulink Support Package for Arduino Hardware
  Byte Pack - 08 : svdutilitieslib/Byte Pack  datatypes={'single'}  byteAlign=1  blockPlatform=arduinoert
      settings: AttributesFormatString=%<datatypes>  SourceProductName=Simulink Support Package for Arduino Hardware
  Byte Pack - 09 : svdutilitieslib/Byte Pack  datatypes={'uint8'}  byteAlign=1  blockPlatform=arduinoert
      settings: AttributesFormatString=%<datatypes>  SourceProductName=Simulink Support Package for Arduino Hardware
  Byte Pack - 10 : svdutilitieslib/Byte Pack  datatypes={'uint8'}  byteAlign=1  blockPlatform=arduinoert
      settings: AttributesFormatString=%<datatypes>  SourceProductName=Simulink Support Package for Arduino Hardware
  Data Type Conversion - 01 : DataTypeConversion  OutDataTypeStr=single
  Data Type Conversion - 02 : DataTypeConversion  OutDataTypeStr=single
  Data Type Conversion - 03 : DataTypeConversion  OutDataTypeStr=single
  Data Type Conversion - 04 : DataTypeConversion  OutDataTypeStr=single
  Data Type Conversion - 05 : DataTypeConversion  OutDataTypeStr=single
  Data Type Conversion - 06 : DataTypeConversion  OutDataTypeStr=single
  Data Type Conversion - 07 : DataTypeConversion  OutDataTypeStr=uint8
  Data Type Conversion - 08 : DataTypeConversion  OutDataTypeStr=uint8
  Data Type Conversion - 09 : DataTypeConversion  OutDataTypeStr=uint8
  Data Type Conversion - 10 : DataTypeConversion  OutDataTypeStr=uint8
  Mux : Mux  Inputs=10
  Rate Transition : RateTransition  X0=io_srl_read_rateTransition_initialCondition  OutPortSampleTimeMultiple=io_read_rateTransition_decimation  OutPortSampleTime=io_srl_read_rateTransition_T_sample
      settings: AttributesFormatString=|
      | Output sample time: %<OutPortSampleTime>
      | Initial condition: %<X0>
  Serial Transmit : arduinolib/Serial Transmit  portNumber=0  sendmode=write  sendformat=Decimal  floatprecision=2  blockPlatform=arduino
      settings: SourceProductName=Simulink Support Package for Arduino Hardware
  wires:
  Bus Selector/1 -> Data Type Conversion - 01/1  "<time [s]>"
  Rate Transition/1 -> Serial Transmit/1
  Bus Selector/4 -> Data Type Conversion - 04/1  "<angularVelocity  [rad/s]>"
  Bus Selector/3 -> Data Type Conversion - 03/1  "<angularVelocity  [rad/s]>"
  Data Type Conversion - 10/1 -> Byte Pack - 10/1
  Data Type Conversion - 09/1 -> Byte Pack - 09/1
  Data Type Conversion - 08/1 -> Byte Pack - 08/1
  Data Type Conversion - 07/1 -> Byte Pack - 07/1
  Data Type Conversion - 06/1 -> Byte Pack - 06/1
  Data Type Conversion - 05/1 -> Byte Pack - 05/1
  Data Type Conversion - 04/1 -> Byte Pack - 04/1
  Data Type Conversion - 03/1 -> Byte Pack - 03/1
  Data Type Conversion - 02/1 -> Byte Pack - 02/1
  Data Type Conversion - 01/1 -> Byte Pack - 01/1
  Byte Pack - 10/1 -> Mux/10
  Byte Pack - 09/1 -> Mux/9
  Bus Selector/2 -> Data Type Conversion - 02/1  "<command>"
  systemSignalBus/1 -> Bus Selector/1
  Byte Pack - 02/1 -> Mux/2
  Byte Pack - 08/1 -> Mux/8
  Byte Pack - 05/1 -> Mux/5
  Byte Pack - 06/1 -> Mux/6
  Byte Pack - 01/1 -> Mux/1
  Mux/1 -> Rate Transition/1
  Byte Pack - 07/1 -> Mux/7
  Byte Pack - 03/1 -> Mux/3
  Byte Pack - 04/1 -> Mux/4
  Bus Selector/5 -> Data Type Conversion - 05/1  "<command [V]>"
  Bus Selector/6 -> Data Type Conversion - 06/1  "<command [V]>"
  Bus Selector/7 -> Data Type Conversion - 07/1  "<positive [V]>"
  Bus Selector/8 -> Data Type Conversion - 08/1  "<negative [V]>"
  Bus Selector/9 -> Data Type Conversion - 09/1  "<positive [V]>"
  Bus Selector/10 -> Data Type Conversion - 10/1  "<negative [V]>"

== system minseg_M2V3_2017a/User IO/Writes (To PC)/Plant: Linear Dynamics/Controller: FF/Standard ==
  systemSignalBus : Inport
  Bus Selector2 : BusSelector  OutputSignals=plant.position.phi.x (pitch).position [rad]
  Bus Selector3 : BusSelector  OutputSignals=controller.output.motorDriver.left.voltage.command [V],controller.output.motorDriver.middle.voltage.command [V]
  pitch : Scope
  v.lm : Scope  NumInputPorts=2
  wires:
  Bus Selector3/1 -> v.lm/1  "<command [V]>"
  systemSignalBus/1 -> Bus Selector3/1, Bus Selector2/1
  Bus Selector3/2 -> v.lm/2  "<command [V]>"
  Bus Selector2/1 -> pitch/1  "<position [rad]>"

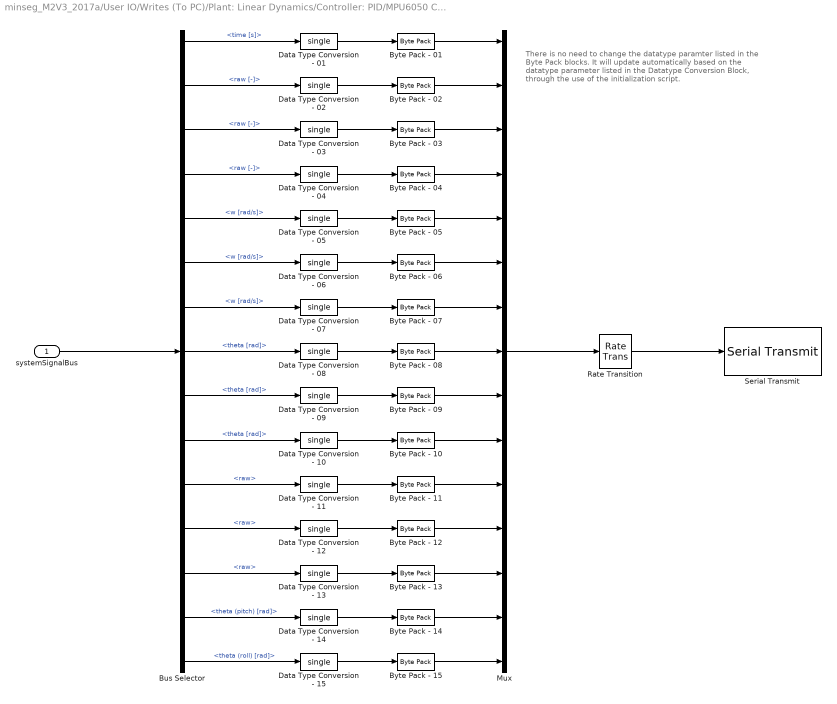
== system minseg_M2V3_2017a/User IO/Writes (To PC)/Plant: Linear Dynamics/Controller: PID/MPU6050 Calibration ==
  note: There is no need to change the datatype paramter
      | listed in the Byte Pack blocks.
      |
      | It will update automatically based on the datatype parameter
      | listed in the Datatype Conversion Block,
      | through the use of the initialization script.
  systemSignalBus : Inport
  Bus Selector : BusSelector  OutputSignals=plant.clock.time [s],plant.gyroscope.x.raw [-],plant.gyroscope.y.raw [-],plant.gyroscope.z.raw [-],plant.gyroscope.x.w [rad/s],plant.gyroscope.y.w [rad/s],plant.gyroscope.z.w [rad/s],plant.gyroscope.x.theta [rad],plant.gyroscope.y.theta [rad],plant.gyroscope.z.theta [rad],plant.accelerometer.x.raw,plant.accelerometer.y.raw,plant.accelerometer.z.raw,plant.accelerometer.x.theta (pitch) [rad],plant.accelerometer.z.theta (roll) [rad]
  Byte Pack - 01 : svdutilitieslib/Byte Pack  datatypes={'single'}  byteAlign=1  blockPlatform=arduinoert
      settings: AttributesFormatString=%<datatypes>  SourceProductName=Simulink Support Package for Arduino Hardware
  Byte Pack - 02 : svdutilitieslib/Byte Pack  datatypes={'single'}  byteAlign=1  blockPlatform=arduinoert
      settings: AttributesFormatString=%<datatypes>  SourceProductName=Simulink Support Package for Arduino Hardware
  Byte Pack - 03 : svdutilitieslib/Byte Pack  datatypes={'single'}  byteAlign=1  blockPlatform=arduinoert
      settings: AttributesFormatString=%<datatypes>  SourceProductName=Simulink Support Package for Arduino Hardware
  Byte Pack - 04 : svdutilitieslib/Byte Pack  datatypes={'single'}  byteAlign=1  blockPlatform=arduinoert
      settings: AttributesFormatString=%<datatypes>  SourceProductName=Simulink Support Package for Arduino Hardware
  Byte Pack - 05 : svdutilitieslib/Byte Pack  datatypes={'single'}  byteAlign=1  blockPlatform=arduinoert
      settings: AttributesFormatString=%<datatypes>  SourceProductName=Simulink Support Package for Arduino Hardware
  Byte Pack - 06 : svdutilitieslib/Byte Pack  datatypes={'single'}  byteAlign=1  blockPlatform=arduinoert
      settings: AttributesFormatString=%<datatypes>  SourceProductName=Simulink Support Package for Arduino Hardware
  Byte Pack - 07 : svdutilitieslib/Byte Pack  datatypes={'single'}  byteAlign=1  blockPlatform=arduinoert
      settings: AttributesFormatString=%<datatypes>  SourceProductName=Simulink Support Package for Arduino Hardware
  Byte Pack - 08 : svdutilitieslib/Byte Pack  datatypes={'single'}  byteAlign=1  blockPlatform=arduinoert
      settings: AttributesFormatString=%<datatypes>  SourceProductName=Simulink Support Package for Arduino Hardware
  Byte Pack - 09 : svdutilitieslib/Byte Pack  datatypes={'single'}  byteAlign=1  blockPlatform=arduinoert
      settings: AttributesFormatString=%<datatypes>  SourceProductName=Simulink Support Package for Arduino Hardware
  Byte Pack - {10..15} (6 alike) : svdutilitieslib/Byte Pack  datatypes={'single'}  byteAlign=1  blockPlatform=arduinoert
      settings: AttributesFormatString=%<datatypes>  SourceProductName=Simulink Support Package for Arduino Hardware
  Data Type Conversion - 01 : DataTypeConversion  OutDataTypeStr=single
  Data Type Conversion - 02 : DataTypeConversion  OutDataTypeStr=single
  Data Type Conversion - 03 : DataTypeConversion  OutDataTypeStr=single
  Data Type Conversion - 04 : DataTypeConversion  OutDataTypeStr=single
  Data Type Conversion - 05 : DataTypeConversion  OutDataTypeStr=single
  Data Type Conversion - 06 : DataTypeConversion  OutDataTypeStr=single
  Data Type Conversion - 07 : DataTypeConversion  OutDataTypeStr=single
  Data Type Conversion - 08 : DataTypeConversion  OutDataTypeStr=single
  Data Type Conversion - 09 : DataTypeConversion  OutDataTypeStr=single
  Data Type Conversion - {10..15} (6 alike) : DataTypeConversion  OutDataTypeStr=single
  Mux : Mux  Inputs=15
  Rate Transition : RateTransition  X0=io_srl_read_rateTransition_initialCondition  OutPortSampleTimeMultiple=io_read_rateTransition_decimation  OutPortSampleTime=io_srl_read_rateTransition_T_sample
      settings: AttributesFormatString=|
      | Output sample time: %<OutPortSampleTime>
      | Initial condition: %<X0>
  Serial Transmit : arduinolib/Serial Transmit  portNumber=0  sendmode=write  sendformat=Decimal  floatprecision=2  blockPlatform=arduino
      settings: SourceProductName=Simulink Support Package for Arduino Hardware
  wires:
  Byte Pack - 04/1 -> Mux/4
  Byte Pack - 03/1 -> Mux/3
  Byte Pack - 07/1 -> Mux/7
  Mux/1 -> Rate Transition/1
  Byte Pack - 01/1 -> Mux/1
  Byte Pack - 06/1 -> Mux/6
  Byte Pack - 05/1 -> Mux/5
  Byte Pack - 08/1 -> Mux/8
  Byte Pack - 02/1 -> Mux/2
  systemSignalBus/1 -> Bus Selector/1
  Byte Pack - 09/1 -> Mux/9
  Byte Pack - 10/1 -> Mux/10
  Data Type Conversion - 01/1 -> Byte Pack - 01/1
  Data Type Conversion - 02/1 -> Byte Pack - 02/1
  Data Type Conversion - 03/1 -> Byte Pack - 03/1
  Data Type Conversion - 04/1 -> Byte Pack - 04/1
  Data Type Conversion - 05/1 -> Byte Pack - 05/1
  Data Type Conversion - 06/1 -> Byte Pack - 06/1
  Data Type Conversion - 07/1 -> Byte Pack - 07/1
  Data Type Conversion - 08/1 -> Byte Pack - 08/1
  Data Type Conversion - 09/1 -> Byte Pack - 09/1
  Data Type Conversion - 10/1 -> Byte Pack - 10/1
  Rate Transition/1 -> Serial Transmit/1
  Bus Selector/1 -> Data Type Conversion - 01/1  "<time [s]>"
  Data Type Conversion - 11/1 -> Byte Pack - 11/1
  Data Type Conversion - 12/1 -> Byte Pack - 12/1
  Data Type Conversion - 13/1 -> Byte Pack - 13/1
  Data Type Conversion - 14/1 -> Byte Pack - 14/1
  Data Type Conversion - 15/1 -> Byte Pack - 15/1
  Byte Pack - 11/1 -> Mux/11
  Byte Pack - 12/1 -> Mux/12
  Byte Pack - 13/1 -> Mux/13
  Byte Pack - 14/1 -> Mux/14
  Byte Pack - 15/1 -> Mux/15
  Bus Selector/2 -> Data Type Conversion - 02/1  "<raw [-]>"
  Bus Selector/3 -> Data Type Conversion - 03/1  "<raw [-]>"
  Bus Selector/4 -> Data Type Conversion - 04/1  "<raw [-]>"
  Bus Selector/5 -> Data Type Conversion - 05/1  "<w [rad/s]>"
  Bus Selector/6 -> Data Type Conversion - 06/1  "<w [rad/s]>"
  Bus Selector/7 -> Data Type Conversion - 07/1  "<w [rad/s]>"
  Bus Selector/8 -> Data Type Conversion - 08/1  "<theta [rad]>"
  Bus Selector/11 -> Data Type Conversion - 11/1  "<raw>"
  Bus Selector/12 -> Data Type Conversion - 12/1  "<raw>"
  Bus Selector/9 -> Data Type Conversion - 09/1  "<theta [rad]>"
  Bus Selector/10 -> Data Type Conversion - 10/1  "<theta [rad]>"
  Bus Selector/13 -> Data Type Conversion - 13/1  "<raw>"
  Bus Selector/14 -> Data Type Conversion - 14/1  "<theta (pitch) [rad]>"
  Bus Selector/15 -> Data Type Conversion - 15/1  "<theta (roll) [rad]>"
